simulink model "gm_sampleModel1830_sub"  (R2023a)
settings: Solver=VariableStepAuto  StartTime=0.0  StopTime=10.0  RelTol=1e-3
libraries: hdlsllib x2, simulink x1
settings Model: Creator=user1  LastModifiedBy=user1
settings OptimizationCC: BlockReduction=off  ConditionallyExecuteInputs=off
settings DebuggingCC: InheritedTsInSrcMsg=none

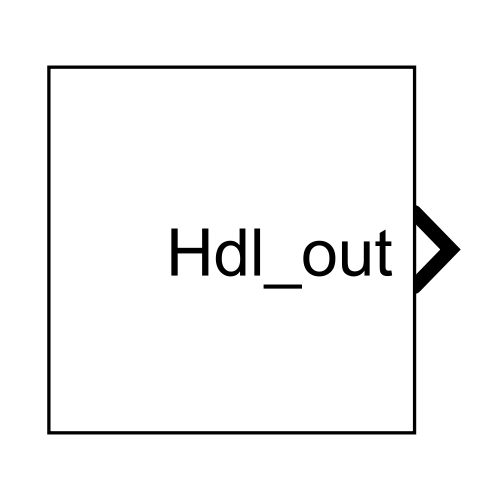
[thumbnail: Simulink's stored preview of the top-level diagram]
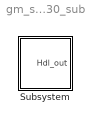
== system gm_sampleModel1830_sub ==
  Subsystem : Subsystem

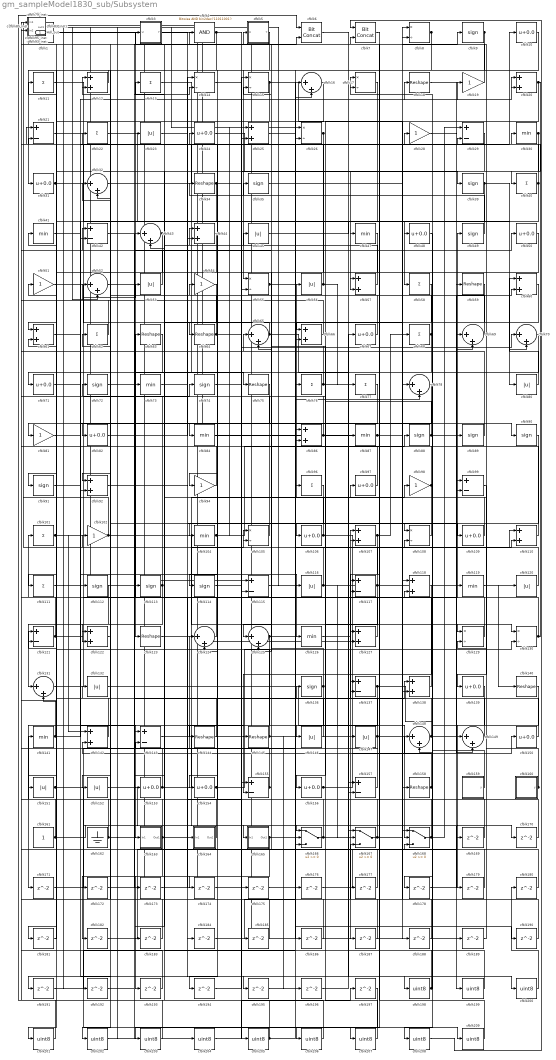
== system gm_sampleModel1830_sub/Subsystem ==
  cfblk1 : RelationalOperator  Operator=<=  OutDataTypeStr=boolean  InputSameDT=off
  cfblk{10,24,31,48,50,67,71,82,97,106,109,139,150,153..154,156} (16 alike) : Bias  Bias=0.0  SaturateOnIntegerOverflow=off
  cfblk100_inst : Subsystem
  cfblk{11,13,22,40,58,62,68,76..77,96,101,111} (12 alike) : Sum  Inputs=+  OutDataTypeStr=uint8
  cfblk{19,28,51,54,81,94,98,102} (8 alike) : Gain  OutDataTypeStr=uint8
  cfblk{30,41,47,73,84,87,104,119,126,141} (10 alike) : MinMax  OutDataTypeStr=uint8
  cfblk{8,14..15,17,26,55,105,108,129..130} (10 alike) : Product  Inputs=*/  OutDataTypeStr=uint8  RndMeth=Zero  SaturateOnIntegerOverflow=on
  cfblk{12,20,25,44,57,60..61,66,86,92,107,110,118,122,127,138,142} (17 alike) : Sum  OutDataTypeStr=uint8
  cfblk{9,35,39,49,72,74,88..91,112..114,136} (14 alike) : Signum
  cfblk{21,29,42,99,115,117,121,137,143,155,157} (11 alike) : Sum  Inputs=+-  OutDataTypeStr=uint8
  cfblk{23,45,53,56,80,116,120,132,146..147,151..152} (12 alike) : Abs  OutDataTypeStr=uint8  SaturateOnIntegerOverflow=off
  cfblk{18,34,59,63..64,75,123,140,144..145,158} (11 alike) : Reshape
  cfblk{16,32,43,52,65,69..70,78,124..125,131,148..149} (13 alike) : Sum  Inputs=|++  OutDataTypeStr=uint8
  cfblk128_inst : Subsystem
  cfblk133_inst : Subsystem
  cfblk134_inst : Subsystem
  cfblk135_inst : Subsystem
  cfblk159 : Subsystem  mask(Counter Free-Running){NumBits=double(16), tsamp=double(-1)}
      mask prompts: NumBits "Simulink:masks:NumberOfBits_MP"; tsamp "Simulink:masks:SampleTime_MP"
      mask help: Simulink:masks:CounterFreeRunning_MD
  cfblk160 : Subsystem  mask(Counter Limited){uplimit=double(7), tsamp=double(-1)}
      mask prompts: uplimit "Simulink:masks:UpperLimit_MP"; tsamp "Simulink:masks:SampleTime_MP"
      mask help: Simulink:masks:CounterLimited_MD
      mask init:
      | nbits = double(8);
      | tsamp = double(-1);
      | uplimit = double(7);
  cfblk161 : Constant  OutDataTypeStr=uint8  SampleTime=-1
  cfblk162 : Ground
  cfblk163 : Subsystem
  cfblk164 : Subsystem
  cfblk165 : Subsystem
  cfblk166 : Switch  OutDataTypeStr=uint8  SaturateOnIntegerOverflow=off  InputSameDT=off
  cfblk167 : Switch  OutDataTypeStr=uint8  SaturateOnIntegerOverflow=off  InputSameDT=off
  cfblk168 : Switch  OutDataTypeStr=uint8  SaturateOnIntegerOverflow=off  InputSameDT=off
  cfblk{169..197} (29 alike) : Delay  SampleTime=1
  cfblk{198..209} (12 alike) : DataTypeConversion  OutDataTypeStr=uint8  SaturateOnIntegerOverflow=off  RndMeth=Floor
  cfblk2 : Constant  Value=0  OutDataTypeStr=uint8  SampleTime=1
  cfblk27_inst : Subsystem
  cfblk3 : Subsystem  mask(Detect Rise Positive){vinit=double(0), InputProcessing=Elements as channels (sample based), OutDataTypeStr=uint8}
      mask prompts: vinit "Simulink:masks:InitialCondition_MP"; InputProcessing "Simulink:masks:InputProcessing_MP"; OutDataTypeStr "Simulink:masks:OutputDataType_MP"
      mask help: Simulink:masks:DetectRisePositive_MD
      mask init:
      | InputProcessing = 'Elements as channels (sample based)';
      | OutDataTypeStr = 'uint8';
      | vinit = double(0);
      mask TypeOptions InputProcessing: Simulink:masks:ColumnsAsChannelsFrameBased | Simulink:masks:ElementsAsChannelsSampleBased
      mask TypeOptions OutDataTypeStr: Simulink:masks:uint8 | Simulink:masks:boolean
      mask Display: fprintf('U > 0\n&  NOT\nU/z > 0')
  cfblk33_inst : Subsystem
  cfblk37_inst : Subsystem
  cfblk4 : simulink/Logic and Bit Operations/Bitwise Operator  logicop=AND  UseBitMask=on  BitMask=bin2dec('11011001')  BitMaskRealWorld=Stored Integer
      settings: LibrarySourceBlock=|
      | hdlsllib/Logic and Bit
      | Operations/Bitwise
      | Operator
  cfblk5 : Subsystem  mask(Detect Rise Positive){vinit=double(0), InputProcessing=Elements as channels (sample based), OutDataTypeStr=uint8}
      mask prompts: vinit "Simulink:masks:InitialCondition_MP"; InputProcessing "Simulink:masks:InputProcessing_MP"; OutDataTypeStr "Simulink:masks:OutputDataType_MP"
      mask help: Simulink:masks:DetectRisePositive_MD
      mask init:
      | InputProcessing = 'Elements as channels (sample based)';
      | OutDataTypeStr = 'uint8';
      | vinit = double(0);
      mask TypeOptions InputProcessing: Simulink:masks:ColumnsAsChannelsFrameBased | Simulink:masks:ElementsAsChannelsSampleBased
      mask TypeOptions OutDataTypeStr: Simulink:masks:uint8 | Simulink:masks:boolean
      mask Display: fprintf('U > 0\n&  NOT\nU/z > 0')
  cfblk6 : hdlsllib/Logic and Bit Operations/Bit Concat  numInputs=2
  cfblk7 : hdlsllib/Logic and Bit Operations/Bit Concat  numInputs=2
  cfblk79_inst : Subsystem
  cfblk83_inst : Subsystem
  cfblk85_inst : Subsystem
  cfblk93_inst : Subsystem
  cfblk95_inst : Subsystem
  Hdl_out : Outport  OutDataTypeStr=uint8  SampleTime=1
  wires:
  cfblk1/1 -> cfblk123/1
  cfblk10/1 -> cfblk55/1
  cfblk100_inst/1(out1) -> cfblk115/1
  cfblk101/1 -> cfblk53/1, cfblk142/1
  cfblk102/1 -> cfblk93_inst/1(in1), cfblk129/1
  cfblk104/1 -> cfblk88/1, cfblk25/1
  cfblk105/1 -> cfblk85_inst/1(in1)
  cfblk106/1 -> cfblk56/1, cfblk110/2
  cfblk107/1 -> cfblk187/1, cfblk68/1
  cfblk108/1 -> cfblk106/1
  cfblk109/1 -> cfblk43/2
  cfblk11/1 -> cfblk43/1
  cfblk110/1 -> cfblk15/2
  cfblk111/1 -> cfblk74/1
  cfblk112/1 -> cfblk131/1
  cfblk113/1 -> cfblk37_inst/1(in1), cfblk181/1
  cfblk114/1 -> cfblk70/1
  cfblk115/1 -> cfblk126/1
  cfblk116/1 -> cfblk35/1, cfblk167/2
  cfblk117/1 -> cfblk93_inst/2(in2), cfblk146/1
  cfblk118/1 -> cfblk155/2
  cfblk119/1 -> cfblk140/1
  cfblk12/1 -> cfblk31/1
  cfblk120/1 -> cfblk76/1
  cfblk121/1 -> cfblk29/2, cfblk135_inst/1(in1)
  cfblk122/1 -> cfblk191/1
  cfblk123/1 -> cfblk105/1
  cfblk124/1 -> cfblk101/1
  cfblk125/1 -> cfblk78/2, cfblk163/1(In1)
  cfblk126/1 -> cfblk107/1
  cfblk127/1 -> cfblk63/1
  cfblk128_inst/1(out1) -> cfblk52/2, cfblk175/1
  cfblk129/1 -> cfblk49/1
  cfblk13/1 -> cfblk205/1
  cfblk130/1 -> cfblk61/2, cfblk30/1
  cfblk131/1 -> cfblk118/2
  cfblk132/1 -> cfblk168/2
  cfblk133_inst/1(out1) -> cfblk204/1, cfblk26/1
  cfblk134_inst/1(out1) -> cfblk95_inst/2(in2), cfblk164/1(In1)
  cfblk135_inst/1(out1) -> cfblk87/1
  cfblk136/1 -> cfblk42/1, cfblk174/1
  cfblk137/1 -> cfblk208/1, cfblk171/1
  cfblk138/1 -> cfblk17/1
  cfblk139/1 -> cfblk179/1
  cfblk14/1 -> cfblk116/1
  cfblk140/1 -> cfblk148/2
  cfblk141/1 -> cfblk83_inst/2(in2), cfblk28/1
  cfblk142/1 -> cfblk121/1
  cfblk143/1 -> cfblk165/1(In1)
  cfblk144/1 -> cfblk132/1
  cfblk145/1 -> cfblk196/1, cfblk11/1
  cfblk146/1 -> cfblk5/1(U)
  cfblk147/1 -> cfblk143/2, cfblk107/2
  cfblk148/1 -> cfblk72/1, cfblk136/1
  cfblk149/1 -> cfblk24/1
  cfblk15/1 -> cfblk91/1, cfblk188/1
  cfblk150/1 -> cfblk45/1
  cfblk151/1 -> cfblk209/1, cfblk166/1, cfblk16/1
  cfblk152/1 -> cfblk176/1
  cfblk153/1 -> cfblk199/1, cfblk12/1, cfblk98/1
  cfblk154/1 -> cfblk206/1, cfblk130/2
  cfblk155/1 -> cfblk65/2, cfblk100_inst/2(in2)
  cfblk156/1 -> cfblk99/1, cfblk150/1
  cfblk157/1 -> cfblk133_inst/1(in1)
  cfblk158/1 -> cfblk148/1, cfblk142/2
  cfblk159/1(y) -> cfblk17/2
  cfblk16/1 -> cfblk92/1
  cfblk160/1(y) -> cfblk99/2, cfblk4/1
  cfblk161/1 -> cfblk166/2, cfblk141/1
  cfblk162/1 -> cfblk138/1, cfblk51/1
  cfblk163/1(Out1) -> cfblk193/1, cfblk119/1, cfblk41/1
  cfblk164/1(Out1) -> cfblk102/1
  cfblk165/1(Out1) -> cfblk110/1, cfblk182/1
  cfblk166/1 -> cfblk67/1, cfblk27_inst/2(in2)
  cfblk167/1 -> cfblk9/1, cfblk62/1
  cfblk168/1 -> cfblk44/1, cfblk29/1
  cfblk169/1 -> cfblk65/1
  cfblk17/1 -> cfblk57/2
  cfblk170/1 -> cfblk133_inst/2(in2)
  cfblk171/1 -> cfblk124/1
  cfblk172/1 -> cfblk78/1
  cfblk173/1 -> cfblk155/1
  cfblk174/1 -> cfblk168/3
  cfblk175/1 -> cfblk168/1
  cfblk176/1 -> cfblk8/2
  cfblk177/1 -> cfblk1/2
  cfblk178/1 -> cfblk60/2
  cfblk179/1 -> cfblk1/1
  cfblk18/1 -> cfblk69/1
  cfblk180/1 -> cfblk105/2
  cfblk181/1 -> cfblk121/2
  cfblk182/1 -> cfblk69/2
  cfblk183/1 -> cfblk32/2
  cfblk184/1 -> cfblk86/1
  cfblk185/1 -> cfblk131/2
  cfblk186/1 -> cfblk21/2
  cfblk187/1 -> cfblk79_inst/2(in2)
  cfblk188/1 -> cfblk167/3
  cfblk189/1 -> cfblk129/2
  cfblk19/1 -> cfblk134_inst/2(in2)
  cfblk190/1 -> cfblk118/1
  cfblk191/1 -> cfblk26/2
  cfblk192/1 -> cfblk14/2
  cfblk193/1 -> cfblk135_inst/2(in2)
  cfblk194/1 -> cfblk55/2
  cfblk195/1 -> cfblk117/2
  cfblk196/1 -> cfblk157/2
  cfblk197/1 -> cfblk203/1
  cfblk198/1 -> cfblk97/1, cfblk108/2
  cfblk199/1 -> cfblk3/1(U)
  cfblk2/1 -> cfblk177/1
  cfblk20/1 -> cfblk66/1, cfblk40/1
  cfblk200/1 -> cfblk180/1
  cfblk201/1 -> cfblk6/1
  cfblk202/1 -> cfblk6/2
  cfblk203/1 -> cfblk85_inst/2(in2)
  cfblk204/1 -> cfblk197/1
  cfblk205/1 -> cfblk16/2, cfblk128_inst/1(in1)
  cfblk206/1 -> cfblk13/1
  cfblk207/1 -> cfblk96/1
  cfblk208/1 -> cfblk7/1
  cfblk209/1 -> cfblk7/2
  cfblk21/1 -> cfblk80/1
  cfblk22/1 -> cfblk58/1
  cfblk23/1 -> cfblk145/1
  cfblk24/1 -> cfblk89/1
  cfblk25/1 -> cfblk190/1
  cfblk26/1 -> cfblk125/1, cfblk124/2
  cfblk27_inst/1(out1) -> cfblk37_inst/2(in2), cfblk33_inst/2(in2)
  cfblk28/1 -> cfblk59/1
  cfblk29/1 -> cfblk73/1
  cfblk3/1(Y) -> cfblk198/1
  cfblk30/1 -> cfblk61/1, cfblk47/1
  cfblk31/1 -> cfblk186/1, cfblk185/1, cfblk184/1
  cfblk32/1 -> cfblk10/1
  cfblk33_inst/1(out1) -> cfblk192/1
  cfblk34/1 -> cfblk71/1, cfblk42/2, cfblk169/1
  cfblk35/1 -> cfblk8/1
  cfblk37_inst/1(out1) -> cfblk147/1
  cfblk39/1 -> cfblk70/2, cfblk154/1
  cfblk4/1 -> cfblk44/2, cfblk39/1, cfblk111/1
  cfblk40/1 -> cfblk202/1, cfblk14/1
  cfblk41/1 -> cfblk90/1
  cfblk42/1 -> cfblk173/1
  cfblk43/1 -> cfblk122/2, cfblk81/1
  cfblk44/1 -> cfblk92/2
  cfblk45/1 -> cfblk48/1
  cfblk47/1 -> cfblk114/1
  cfblk48/1 -> cfblk178/1
  cfblk49/1 -> cfblk34/1
  cfblk5/1(Y) -> cfblk194/1
  cfblk50/1 -> cfblk137/2
  cfblk51/1 -> cfblk158/1
  cfblk52/1 -> cfblk50/1
  cfblk53/1 -> cfblk33_inst/1(in1)
  cfblk54/1 -> cfblk153/1
  cfblk55/1 -> cfblk125/2, cfblk170/1
  cfblk56/1 -> cfblk79_inst/1(in1), cfblk77/1
  cfblk57/1 -> cfblk21/1
  cfblk58/1 -> cfblk156/1
  cfblk59/1 -> cfblk138/2
  cfblk6/1 -> cfblk200/1
  cfblk60/1 -> cfblk86/2
  cfblk61/1 -> cfblk143/1
  cfblk62/1 -> cfblk95_inst/1(in1)
  cfblk63/1 -> cfblk151/1
  cfblk64/1 -> cfblk25/2, cfblk134_inst/1(in1), cfblk84/1
  cfblk65/1 -> cfblk64/1, cfblk157/1
  cfblk66/1 -> cfblk52/1
  cfblk67/1 -> cfblk15/1
  cfblk68/1 -> cfblk12/2, cfblk183/1
  cfblk69/1 -> cfblk32/1
  cfblk7/1 -> cfblk207/1
  cfblk70/1 -> cfblk144/1
  cfblk71/1 -> cfblk18/1
  cfblk72/1 -> cfblk75/1
  cfblk73/1 -> cfblk19/1
  cfblk74/1 -> cfblk127/1
  cfblk75/1 -> cfblk82/1
  cfblk76/1 -> cfblk54/1, cfblk108/1
  cfblk77/1 -> cfblk201/1
  cfblk78/1 -> cfblk137/1
  cfblk79_inst/1(out1) -> cfblk113/1, cfblk189/1
  cfblk8/1 -> cfblk57/1, cfblk166/3
  cfblk80/1 -> cfblk60/1
  cfblk81/1 -> cfblk195/1
  cfblk82/1 -> cfblk20/1
  cfblk83_inst/1(out1) -> cfblk149/1
  cfblk84/1 -> cfblk20/2
  cfblk85_inst/1(out1) -> cfblk112/1
  cfblk86/1 -> cfblk167/1, cfblk128_inst/2(in2)
  cfblk87/1 -> cfblk130/1, Hdl_out/1
  cfblk88/1 -> cfblk66/2, cfblk149/2
  cfblk89/1 -> cfblk100_inst/1(in1)
  cfblk9/1 -> cfblk152/1, cfblk94/1
  cfblk90/1 -> cfblk117/1
  cfblk91/1 -> cfblk115/2
  cfblk92/1 -> cfblk109/1
  cfblk93_inst/1(out1) -> cfblk23/1, cfblk127/2
  cfblk94/1 -> cfblk22/1
  cfblk95_inst/1(out1) -> cfblk120/1
  cfblk96/1 -> cfblk172/1
  cfblk97/1 -> cfblk27_inst/1(in1)
  cfblk98/1 -> cfblk83_inst/1(in1), cfblk122/1, cfblk104/1
  cfblk99/1 -> cfblk139/1

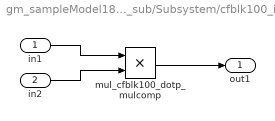
== system gm_sampleModel1830_sub/Subsystem/cfblk100_inst ==
  in1 : Inport  OutDataTypeStr=uint8  SampleTime=1
  in2 : Inport  Port=2  OutDataTypeStr=uint8  SampleTime=1
  mul_cfblk100_dotp_mulcomp : Product  Inputs=**  OutDataTypeStr=uint8  SampleTime=1
  out1 : Outport  OutDataTypeStr=uint8  SampleTime=1
  wires:
  in1/1 -> mul_cfblk100_dotp_mulcomp/1
  in2/1 -> mul_cfblk100_dotp_mulcomp/2
  mul_cfblk100_dotp_mulcomp/1 -> out1/1

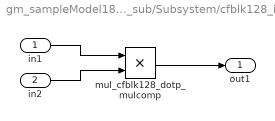
== system gm_sampleModel1830_sub/Subsystem/cfblk128_inst ==
  in1 : Inport  OutDataTypeStr=uint8  SampleTime=1
  in2 : Inport  Port=2  OutDataTypeStr=uint8  SampleTime=1
  mul_cfblk128_dotp_mulcomp : Product  Inputs=**  OutDataTypeStr=uint8  SampleTime=1
  out1 : Outport  OutDataTypeStr=uint8  SampleTime=1
  wires:
  in1/1 -> mul_cfblk128_dotp_mulcomp/1
  in2/1 -> mul_cfblk128_dotp_mulcomp/2
  mul_cfblk128_dotp_mulcomp/1 -> out1/1

== system gm_sampleModel1830_sub/Subsystem/cfblk133_inst ==
  in1 : Inport  OutDataTypeStr=uint8  SampleTime=1
  in2 : Inport  Port=2  OutDataTypeStr=uint8  SampleTime=1
  mul_cfblk133_dotp_mulcomp : Product  Inputs=**  OutDataTypeStr=uint8  SampleTime=1
  out1 : Outport  OutDataTypeStr=uint8  SampleTime=1
  wires:
  in1/1 -> mul_cfblk133_dotp_mulcomp/1
  in2/1 -> mul_cfblk133_dotp_mulcomp/2
  mul_cfblk133_dotp_mulcomp/1 -> out1/1

== system gm_sampleModel1830_sub/Subsystem/cfblk134_inst ==
  in1 : Inport  OutDataTypeStr=uint8  SampleTime=1
  in2 : Inport  Port=2  OutDataTypeStr=uint8  SampleTime=1
  mul_cfblk134_dotp_mulcomp : Product  Inputs=**  OutDataTypeStr=uint8  SampleTime=1
  out1 : Outport  OutDataTypeStr=uint8  SampleTime=1
  wires:
  in1/1 -> mul_cfblk134_dotp_mulcomp/1
  in2/1 -> mul_cfblk134_dotp_mulcomp/2
  mul_cfblk134_dotp_mulcomp/1 -> out1/1

== system gm_sampleModel1830_sub/Subsystem/cfblk135_inst ==
  in1 : Inport  OutDataTypeStr=uint8  SampleTime=1
  in2 : Inport  Port=2  OutDataTypeStr=uint8  SampleTime=1
  mul_cfblk135_dotp_mulcomp : Product  Inputs=**  OutDataTypeStr=uint8  SampleTime=1
  out1 : Outport  OutDataTypeStr=uint8  SampleTime=1
  wires:
  in1/1 -> mul_cfblk135_dotp_mulcomp/1
  in2/1 -> mul_cfblk135_dotp_mulcomp/2
  mul_cfblk135_dotp_mulcomp/1 -> out1/1

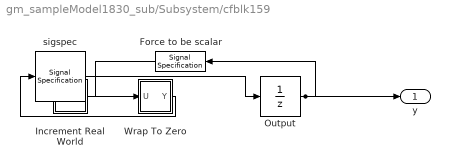
== system gm_sampleModel1830_sub/Subsystem/cfblk159 ==
  Force to be scalar : SignalSpecification  DisableCoverage=on  Dimensions=1
  Increment Real World : Subsystem  mask(Real World Value Increment){}
      mask help: Simulink:masks:RealWorldValueIncrement_MD
      mask Display: disp('V++')
  Output : UnitDelay  InitialCondition=0.0  SampleTime=tsamp  HasFrameUpgradeWarning=on
  Wrap To Zero : Subsystem  mask(Wrap To Zero){Threshold=double(65535)}
      mask prompts: Threshold "Simulink:masks:Threshold_MP"
      mask help: Simulink:masks:WrapToZero_MD
  sigspec : SignalSpecification  OutDataTypeStr=uint16  Dimensions=1
  y : Outport  SampleTime=1
  wires:
  Force to be scalar/1 -> Increment Real World/1(u)
  Increment Real World/1(y) -> Wrap To Zero/1(U)
  Output/1 -> Force to be scalar/1, y/1
  Wrap To Zero/1(Y) -> sigspec/1
  sigspec/1 -> Output/1

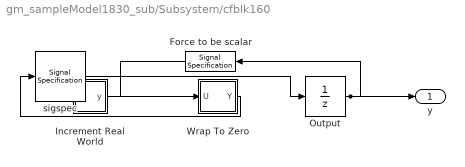
== system gm_sampleModel1830_sub/Subsystem/cfblk160 ==
  Force to be scalar : SignalSpecification  DisableCoverage=on  Dimensions=1
  Increment Real World : Subsystem  mask(Real World Value Increment){}
      mask help: Simulink:masks:RealWorldValueIncrement_MD
      mask Display: disp('V++')
  Output : UnitDelay  InitialCondition=0.0  SampleTime=tsamp  HasFrameUpgradeWarning=on
  Wrap To Zero : Subsystem  mask(Wrap To Zero){Threshold=double(7)}
      mask prompts: Threshold "Simulink:masks:Threshold_MP"
      mask help: Simulink:masks:WrapToZero_MD
  sigspec : SignalSpecification  OutDataTypeStr=uint8  Dimensions=1
  y : Outport  SampleTime=1
  wires:
  Force to be scalar/1 -> Increment Real World/1(u)
  Increment Real World/1(y) -> Wrap To Zero/1(U)
  Output/1 -> Force to be scalar/1, y/1
  Wrap To Zero/1(Y) -> sigspec/1
  sigspec/1 -> Output/1

== system gm_sampleModel1830_sub/Subsystem/cfblk163 ==
  In1 : Inport  OutDataTypeStr=uint8  PortDimensions=1  SampleTime=1
  Out1 : Outport  SampleTime=1
  wires:
  In1/1 -> Out1/1

== system gm_sampleModel1830_sub/Subsystem/cfblk164 ==
  In1 : Inport  OutDataTypeStr=uint8  PortDimensions=1  SampleTime=1
  Out1 : Outport  SampleTime=1
  wires:
  In1/1 -> Out1/1

== system gm_sampleModel1830_sub/Subsystem/cfblk165 ==
  In1 : Inport  OutDataTypeStr=uint8  PortDimensions=1  SampleTime=1
  Out1 : Outport  SampleTime=1
  wires:
  In1/1 -> Out1/1

== system gm_sampleModel1830_sub/Subsystem/cfblk27_inst ==
  in1 : Inport  OutDataTypeStr=uint8  SampleTime=1
  in2 : Inport  Port=2  OutDataTypeStr=uint8  SampleTime=1
  mul_cfblk27_dotp_mulcomp : Product  Inputs=**  OutDataTypeStr=uint8  SampleTime=1
  out1 : Outport  OutDataTypeStr=uint8  SampleTime=1
  wires:
  in1/1 -> mul_cfblk27_dotp_mulcomp/1
  in2/1 -> mul_cfblk27_dotp_mulcomp/2
  mul_cfblk27_dotp_mulcomp/1 -> out1/1

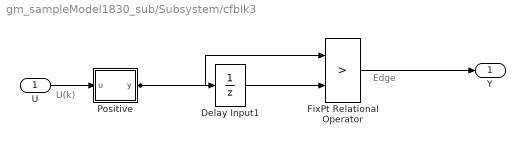
== system gm_sampleModel1830_sub/Subsystem/cfblk3 ==
  note: U(k)
  note: Edge
  U : Inport  OutDataTypeStr=uint8  SampleTime=1
  Delay Input1 : UnitDelay  Description=Store in Global RAM  DisableCoverage=on  InitialCondition=vinit  SampleTime=-1  HasFrameUpgradeWarning=on
  FixPt Relational Operator : RelationalOperator  Operator=>  OutDataTypeStr=fixdt(0, 8)  ZeroCross=off  InputSameDT=off
  Positive : Subsystem  mask(Compare To Zero){relop=>, OutDataTypeStr=boolean, ZeroCross=off}
      mask prompts: relop "Simulink:masks:Operator_MP"; OutDataTypeStr "Simulink:masks:OutputDataType_MP"; ZeroCross "Simulink:masks:EnableZerocrossingDetection_MP"
      mask help: Simulink:masks:CompareToZero_MD
      mask init:
      | OutDataTypeStr = 'boolean';
      | ZeroCross = 'off';
      | blkName = 'sampleModel1830_sub/Subsystem/cfblk3/Positive';
      | relop = '>';
      | setValue = 'boolean';
      mask TypeOptions relop: == | ~= | < | <= | >= | >
      mask TypeOptions OutDataTypeStr: Simulink:masks:uint8 | Simulink:masks:boolean
      mask Callback ZeroCross: sl('zeroCrossEnable', gcbh);
      mask Display: disp([relop,' 0'])
  Y : Outport  SampleTime=1
  wires:
  U/1 -> Positive/1(u)
  Delay Input1/1 -> FixPt Relational Operator/2
  FixPt Relational Operator/1 -> Y/1
  Positive/1(y) -> FixPt Relational Operator/1, Delay Input1/1

== system gm_sampleModel1830_sub/Subsystem/cfblk33_inst ==
  in1 : Inport  OutDataTypeStr=uint8  SampleTime=1
  in2 : Inport  Port=2  OutDataTypeStr=uint8  SampleTime=1
  mul_cfblk33_dotp_mulcomp : Product  Inputs=**  OutDataTypeStr=uint8  SampleTime=1
  out1 : Outport  OutDataTypeStr=uint8  SampleTime=1
  wires:
  in1/1 -> mul_cfblk33_dotp_mulcomp/1
  in2/1 -> mul_cfblk33_dotp_mulcomp/2
  mul_cfblk33_dotp_mulcomp/1 -> out1/1

== system gm_sampleModel1830_sub/Subsystem/cfblk37_inst ==
  in1 : Inport  OutDataTypeStr=uint8  SampleTime=1
  in2 : Inport  Port=2  OutDataTypeStr=uint8  SampleTime=1
  mul_cfblk37_dotp_mulcomp : Product  Inputs=**  OutDataTypeStr=uint8  SampleTime=1
  out1 : Outport  OutDataTypeStr=uint8  SampleTime=1
  wires:
  in1/1 -> mul_cfblk37_dotp_mulcomp/1
  in2/1 -> mul_cfblk37_dotp_mulcomp/2
  mul_cfblk37_dotp_mulcomp/1 -> out1/1

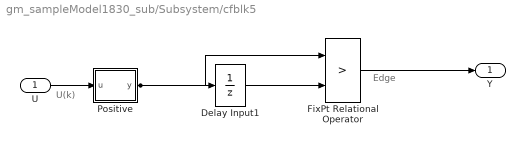
== system gm_sampleModel1830_sub/Subsystem/cfblk5 ==
  note: U(k)
  note: Edge
  U : Inport  OutDataTypeStr=uint8  SampleTime=1
  Delay Input1 : UnitDelay  Description=Store in Global RAM  DisableCoverage=on  InitialCondition=vinit  SampleTime=-1  HasFrameUpgradeWarning=on
  FixPt Relational Operator : RelationalOperator  Operator=>  OutDataTypeStr=fixdt(0, 8)  ZeroCross=off  InputSameDT=off
  Positive : Subsystem  mask(Compare To Zero){relop=>, OutDataTypeStr=boolean, ZeroCross=off}
      mask prompts: relop "Simulink:masks:Operator_MP"; OutDataTypeStr "Simulink:masks:OutputDataType_MP"; ZeroCross "Simulink:masks:EnableZerocrossingDetection_MP"
      mask help: Simulink:masks:CompareToZero_MD
      mask init:
      | OutDataTypeStr = 'boolean';
      | ZeroCross = 'off';
      | blkName = 'sampleModel1830_sub/Subsystem/cfblk5/Positive';
      | relop = '>';
      | setValue = 'boolean';
      mask TypeOptions relop: == | ~= | < | <= | >= | >
      mask TypeOptions OutDataTypeStr: Simulink:masks:uint8 | Simulink:masks:boolean
      mask Callback ZeroCross: sl('zeroCrossEnable', gcbh);
      mask Display: disp([relop,' 0'])
  Y : Outport  SampleTime=1
  wires:
  U/1 -> Positive/1(u)
  Delay Input1/1 -> FixPt Relational Operator/2
  FixPt Relational Operator/1 -> Y/1
  Positive/1(y) -> FixPt Relational Operator/1, Delay Input1/1

== system gm_sampleModel1830_sub/Subsystem/cfblk79_inst ==
  in1 : Inport  OutDataTypeStr=uint8  SampleTime=1
  in2 : Inport  Port=2  OutDataTypeStr=uint8  SampleTime=1
  mul_cfblk79_dotp_mulcomp : Product  Inputs=**  OutDataTypeStr=uint8  SampleTime=1
  out1 : Outport  OutDataTypeStr=uint8  SampleTime=1
  wires:
  in1/1 -> mul_cfblk79_dotp_mulcomp/1
  in2/1 -> mul_cfblk79_dotp_mulcomp/2
  mul_cfblk79_dotp_mulcomp/1 -> out1/1

== system gm_sampleModel1830_sub/Subsystem/cfblk83_inst ==
  in1 : Inport  OutDataTypeStr=uint8  SampleTime=1
  in2 : Inport  Port=2  OutDataTypeStr=uint8  SampleTime=1
  mul_cfblk83_dotp_mulcomp : Product  Inputs=**  OutDataTypeStr=uint8  SampleTime=1
  out1 : Outport  OutDataTypeStr=uint8  SampleTime=1
  wires:
  in1/1 -> mul_cfblk83_dotp_mulcomp/1
  in2/1 -> mul_cfblk83_dotp_mulcomp/2
  mul_cfblk83_dotp_mulcomp/1 -> out1/1

== system gm_sampleModel1830_sub/Subsystem/cfblk85_inst ==
  in1 : Inport  OutDataTypeStr=uint8  SampleTime=1
  in2 : Inport  Port=2  OutDataTypeStr=uint8  SampleTime=1
  mul_cfblk85_dotp_mulcomp : Product  Inputs=**  OutDataTypeStr=uint8  SampleTime=1
  out1 : Outport  OutDataTypeStr=uint8  SampleTime=1
  wires:
  in1/1 -> mul_cfblk85_dotp_mulcomp/1
  in2/1 -> mul_cfblk85_dotp_mulcomp/2
  mul_cfblk85_dotp_mulcomp/1 -> out1/1

== system gm_sampleModel1830_sub/Subsystem/cfblk93_inst ==
  in1 : Inport  OutDataTypeStr=uint8  SampleTime=1
  in2 : Inport  Port=2  OutDataTypeStr=uint8  SampleTime=1
  mul_cfblk93_dotp_mulcomp : Product  Inputs=**  OutDataTypeStr=uint8  SampleTime=1
  out1 : Outport  OutDataTypeStr=uint8  SampleTime=1
  wires:
  in1/1 -> mul_cfblk93_dotp_mulcomp/1
  in2/1 -> mul_cfblk93_dotp_mulcomp/2
  mul_cfblk93_dotp_mulcomp/1 -> out1/1

== system gm_sampleModel1830_sub/Subsystem/cfblk95_inst ==
  in1 : Inport  OutDataTypeStr=uint8  SampleTime=1
  in2 : Inport  Port=2  OutDataTypeStr=uint8  SampleTime=1
  mul_cfblk95_dotp_mulcomp : Product  Inputs=**  OutDataTypeStr=uint8  SampleTime=1
  out1 : Outport  OutDataTypeStr=uint8  SampleTime=1
  wires:
  in1/1 -> mul_cfblk95_dotp_mulcomp/1
  in2/1 -> mul_cfblk95_dotp_mulcomp/2
  mul_cfblk95_dotp_mulcomp/1 -> out1/1

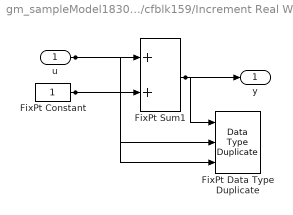
== system gm_sampleModel1830_sub/Subsystem/cfblk159/Increment Real World ==
  u : Inport  OutDataTypeStr=uint16  SampleTime=1
  FixPt Constant : Constant  DisableCoverage=on  OutDataTypeStr=Inherit: Inherit via back propagation  SampleTime=-1
  FixPt Data Type Duplicate : DataTypeDuplicate  DisableCoverage=on  NumInputPorts=3
  FixPt Sum1 : Sum  InputSameDT=on  OutDataTypeStr=Inherit: Inherit via back propagation  LockScale=on
  y : Outport  SampleTime=1
  wires:
  u/1 -> FixPt Sum1/1, FixPt Data Type Duplicate/2
  FixPt Constant/1 -> FixPt Sum1/2, FixPt Data Type Duplicate/3
  FixPt Sum1/1 -> FixPt Data Type Duplicate/1, y/1

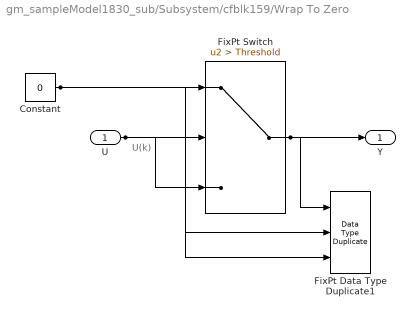
== system gm_sampleModel1830_sub/Subsystem/cfblk159/Wrap To Zero ==
  note: U(k)
  U : Inport  OutDataTypeStr=uint16  SampleTime=1
  Constant : Constant  DisableCoverage=on  Value=0  OutDataTypeStr=Inherit: Inherit via back propagation  SampleTime=-1
  FixPt Data Type Duplicate1 : DataTypeDuplicate  DisableCoverage=on  NumInputPorts=3
  FixPt Switch : Switch  Criteria=u2 > Threshold  Threshold=Threshold  OutDataTypeStr=Inherit: Inherit via back propagation  ZeroCross=off  SaturateOnIntegerOverflow=off  InputSameDT=off
  Y : Outport  SampleTime=1
  wires:
  U/1 -> FixPt Switch/3, FixPt Switch/2, FixPt Data Type Duplicate1/2
  Constant/1 -> FixPt Switch/1, FixPt Data Type Duplicate1/3
  FixPt Switch/1 -> FixPt Data Type Duplicate1/1, Y/1

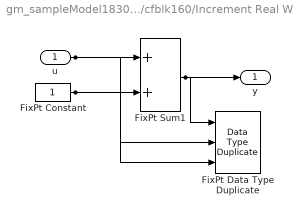
== system gm_sampleModel1830_sub/Subsystem/cfblk160/Increment Real World ==
  u : Inport  OutDataTypeStr=uint8  SampleTime=1
  FixPt Constant : Constant  DisableCoverage=on  OutDataTypeStr=Inherit: Inherit via back propagation  SampleTime=-1
  FixPt Data Type Duplicate : DataTypeDuplicate  DisableCoverage=on  NumInputPorts=3
  FixPt Sum1 : Sum  InputSameDT=on  OutDataTypeStr=Inherit: Inherit via back propagation  LockScale=on
  y : Outport  SampleTime=1
  wires:
  u/1 -> FixPt Sum1/1, FixPt Data Type Duplicate/2
  FixPt Constant/1 -> FixPt Sum1/2, FixPt Data Type Duplicate/3
  FixPt Sum1/1 -> FixPt Data Type Duplicate/1, y/1

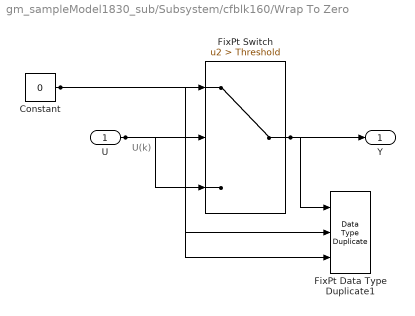
== system gm_sampleModel1830_sub/Subsystem/cfblk160/Wrap To Zero ==
  note: U(k)
  U : Inport  OutDataTypeStr=uint8  SampleTime=1
  Constant : Constant  DisableCoverage=on  Value=0  OutDataTypeStr=Inherit: Inherit via back propagation  SampleTime=-1
  FixPt Data Type Duplicate1 : DataTypeDuplicate  DisableCoverage=on  NumInputPorts=3
  FixPt Switch : Switch  Criteria=u2 > Threshold  Threshold=Threshold  OutDataTypeStr=Inherit: Inherit via back propagation  ZeroCross=off  SaturateOnIntegerOverflow=off  InputSameDT=off
  Y : Outport  SampleTime=1
  wires:
  U/1 -> FixPt Switch/3, FixPt Switch/2, FixPt Data Type Duplicate1/2
  Constant/1 -> FixPt Switch/1, FixPt Data Type Duplicate1/3
  FixPt Switch/1 -> FixPt Data Type Duplicate1/1, Y/1

== system gm_sampleModel1830_sub/Subsystem/cfblk3/Positive ==
  u : Inport  OutDataTypeStr=uint8  SampleTime=1
  Compare : RelationalOperator  Operator=>  OutDataTypeStr=boolean  ZeroCross=off
  Constant : Constant  DisableCoverage=on  Value=0  OutDataTypeStr=Inherit: Inherit via back propagation  SampleTime=-1  PreserveConstantTs=on
  y : Outport  SampleTime=1
  wires:
  u/1 -> Compare/1
  Compare/1 -> y/1
  Constant/1 -> Compare/2

== system gm_sampleModel1830_sub/Subsystem/cfblk5/Positive ==
  u : Inport  OutDataTypeStr=uint8  SampleTime=1
  Compare : RelationalOperator  Operator=>  OutDataTypeStr=boolean  ZeroCross=off
  Constant : Constant  DisableCoverage=on  Value=0  OutDataTypeStr=Inherit: Inherit via back propagation  SampleTime=-1  PreserveConstantTs=on
  y : Outport  SampleTime=1
  wires:
  u/1 -> Compare/1
  Compare/1 -> y/1
  Constant/1 -> Compare/2
